simulink model "Shaft_TestBed"  (R2019b)
settings: Solver=FixedStepDiscrete  StartTime=0.0  StopTime=1  FixedStep=1  RelTol=1e-3  EnableMultiTasking=on
undefined symbols (not defined in the file): MWS
libraries: Lib_Turbo_Shaft_TMATS x1
settings Model: Creator=jwchapm2  LastModifiedBy=bhisma
settings DataIOCC: LimitDataPoints=on  SaveFormat=Array  ReturnWorkspaceOutputs=off
settings OptimizationCC: ExpressionDepthLimit=2147483647  LifeSpan=inf
settings DebuggingCC: UnderspecifiedInitializationDetection=Classic  MergeDetectMultiDrivingBlocksExec=none  SolverPrmCheckMsg=warning  StateNameClashWarn=warning  SFUnexpectedBacktrackingDiag=warning  SFNoUnconditionalDefaultTransitionDiag=warning  SFExecutionAtInitializationDiag=none  ArithmeticOperatorsInVariantConditions=warning
settings HardwareCC: ProdBitPerPointer=32  ProdBitPerSizeT=32  ProdBitPerPtrDiffT=32  ProdLargestAtomicFloat=None  ProdIntDivRoundTo=Undefined  ProdEndianess=Unspecified  ProdWordSize=32  ProdHWDeviceType=32-bit Generic
settings ModelReferenceCC: PropagateSignalLabelsOutOfModel=off
settings SFSimCC: SimUseLocalCustomCode=off  CustomCodeUndefinedFunction=UseInterfaceOnly
settings RTWCC: RTWUseLocalCustomCode=off
settings CodeAppCC: StateflowObjectComments=on
settings GRTTargetCC: TargetLangStandard=C89/C90 (ANSI)  GeneratePreprocessorConditionals=Disable all
settings ConfigComp: CovMetricSettings=dw  CovHtmlReporting=on  CovSaveCumulativeToWorkspaceVar=on  CovSaveSingleToWorkspaceVar=on  CovExternalEMLEnable=off

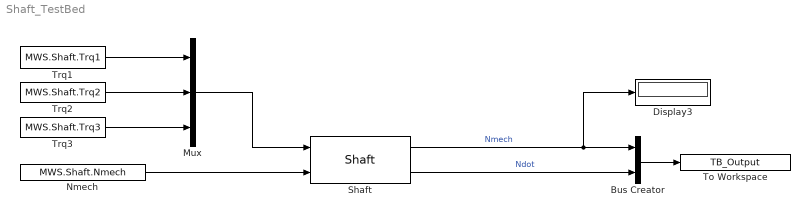
== system Shaft_TestBed ==
  Bus Creator : BusCreator  Inputs=2
  Display3 : Display
  Mux : Mux  Inputs=3
  Nmech : Constant  Value=MWS.Shaft.Nmech
  Shaft : Lib_Turbo_Shaft_TMATS/Shaft  Shaft_Inertia_M=MWS.Shaft.Inertia
  To Workspace : ToWorkspace  VariableName=TB_Output  SampleTime=-1
  Trq1 : Constant  Value=MWS.Shaft.Trq1
  Trq2 : Constant  Value=MWS.Shaft.Trq2
  Trq3 : Constant  Value=MWS.Shaft.Trq3
  wires:
  Trq1/1 -> Mux/1
  Nmech/1 -> Shaft/2
  Trq3/1 -> Mux/3
  Shaft/1 -> Display3/1, Bus Creator/1  "Nmech"
  Bus Creator/1 -> To Workspace/1
  Trq2/1 -> Mux/2
  Mux/1 -> Shaft/1
  Shaft/2 -> Bus Creator/2  "Ndot"
